simulink model "Basic_DMT"  (R2014b)
settings: Solver=FixedStepDiscrete  SolverMode=SingleTasking  StartTime=0.0  StopTime=25e-6-14e-9*24  RelTol=1e-3
PreLoadFcn:
  | userName = getenv('UserName');
  | 
  | if strcmp(userName,'Tim')
  | cd C:\Users\Tim\Documents\GitHub\MA_1\Basic_DMT
  | else
  | cd C:\Users\Tim-UML\Documents\GitHub\MA_1\Basic_DMT
  | end
InitFcn:
  | userName = getenv('UserName');
  | 
  | if strcmp(userName,'Tim')
  | cd C:\Users\Tim\Documents\GitHub\MA_1\Basic_DMT
  | else
  | cd C:\Users\Tim-UML\Documents\GitHub\MA_1\Basic_DMT
  | end
values from neighbouring files (symbols this model uses):
  a0 = 0.21194908595403703    (= 0.211949085954)    [initScript.m]
  a1 = 0.576101828091926    (= 0.576101828092)    [initScript.m]
  a2 = a0    (= 0.211949085954)    [initScript.m]
  beta = 1    [initScript.m]
  bitPerSymb = 4    [initScript.m]
  chanDownFact = Tchan/SystemPeriod    [initScript.m]
  fftLen = 16    [initScript.m]
  fftLenActive = fftLenDMT    (= 32)    [initScript.m]
  fftLenDMT = 2*fftLen    (= 32)    [initScript.m]
  GI_Active = GI_LenDMT    (= 0)    [initScript.m]
  GI_Len = 0    [initScript.m]
  GI_LenDMT = 0    [initScript.m]
  M = log2(fftLen)    [initScript.m]
  sysgenSystemPeriod = 4e-9    (= 4e-09)    [initScript.m]
  SystemPeriod = 4e-9    (= 4e-09)    [initScript.m]
  upsampleFactor = 1    [initScript.m]
  usedSubCar = 14    [initScript.m]
undefined symbols (not defined in the file or in its folder): bitCount, get, modu_mode, Tb, Ts
libraries: xbsIndex_r4 x822, commdigbbndam3 x59, simulink x42, dspsigops x7, commrandsrc2 x6, dspbuff3 x4, dspxfrm3 x3, dspswit3 x2, commseqgen2 x1, dsparch4 x1, commutil2 x1, dspsnks4 x1
(part 5 of 10)

== system Basic_DMT/Sysgen_AWGN/Yes_AWGN ==
  Re : Inport
  Im : Inport  Port=2
  AddSub : xbsIndex_r4/AddSub  mode=Subtraction  use_carryin=off  use_carryout=off  en=off  latency=1  precision=User Defined  arith_type="Signed  (2's comp)"  n_bits=bitCount+(log2(fftLen)+1)  bin_pt=fracLen  quantization="Round  (unbiased: +/- Inf)"  overflow=Saturate  use_behavioral_HDL=off  hw_selection=Fabric  pipelined=off  dbl_ovrd=off  block_type=addsub
  AddSub1 : xbsIndex_r4/AddSub  mode=Addition  use_carryin=off  use_carryout=off  en=off  latency=0  precision=User Defined  arith_type="Signed  (2's comp)"  n_bits=bitCount+(log2(fftLen)+1)  bin_pt=fracLen  quantization="Round  (unbiased: +/- Inf)"  overflow=Saturate  use_behavioral_HDL=off  hw_selection=Fabric  pipelined=off  dbl_ovrd=off  block_type=addsub
  AddSub2 : xbsIndex_r4/AddSub  mode=Addition  use_carryin=off  use_carryout=off  en=off  latency=0  precision=User Defined  arith_type="Signed  (2's comp)"  n_bits=bitCount+(log2(fftLen)+1)  bin_pt=fracLen  quantization="Round  (unbiased: +/- Inf)"  overflow=Saturate  use_behavioral_HDL=off  hw_selection=Fabric  pipelined=off  dbl_ovrd=off  block_type=addsub
  Assert : xbsIndex_r4/Assert  assert_type=on  type_source=Explicitly  gui_display_data_type=Boolean  arith_type=Boolean  n_bits=16  bin_pt=14  preci_type=Single  exp_width=8  frac_width=24  assert_rate=on  rate_source=Explicitly  period=bitPerSymb*usedSubCar*Ts/(fftLenActive+GI_Active)  output_port=on  block_type=assert
  CMult : xbsIndex_r4/CMult  const=1.58*2  gui_display_data_type=Fixed-point  const_n_bits=bitCount+(log2(fftLen)+1)  const_bin_pt=fracLen  float_type=Single  exp_bits=8  fraction_bits=24  en=off  latency=1  precision=User Defined  arith_type="Signed  (2's comp)"  n_bits=bitCount+(log2(fftLen)+1)  bin_pt=fracLen  quantization="Round  (unbiased: +/- Inf)"  overflow=Saturate  use_behavioral_HDL=off  mem_type=Distributed RAM  pipeline=off  dbl_ovrd=off  block_type=cmult
  Constant1 : xbsIndex_r4/Constant  const=0.5  gui_display_data_type=Fixed-point  arith_type=Signed (2's comp)  n_bits=bitCount+(log2(fftLen)+1)  bin_pt=fracLen  preci_type=Single  exp_width=8  frac_width=24  explicit_period=on  period=bitPerSymb*usedSubCar*Ts/(fftLenActive+GI_Active)  equ=P=C  opselect=C  inp2=PCIN>>17  opr=+  inp1=P  carry=CIN  dbl_ovrd=off  block_type=constant
  Convert : xbsIndex_r4/Convert  gui_display_data_type=Fixed-point  arith_type="Signed  (2's comp)"  n_bits=bitCount+(log2(fftLen)+1)  bin_pt=fracLen  float_type=Single  exp_bits=8  fraction_bits=24  quantization=Truncate  overflow=Wrap  en=off  latency=1  pipeline=off  dbl_ovrd=off  block_type=convert
  Logical : xbsIndex_r4/Logical  logical_function=XOR  inputs=4  en=off  latency=0  precision=Full  arith_type=Unsigned  n_bits=16  bin_pt=0  align_bp=on  dbl_ovrd=off  block_type=logical
  Logical1 : xbsIndex_r4/Logical  logical_function=XOR  inputs=2  en=off  latency=0  precision=Full  arith_type=Unsigned  n_bits=16  bin_pt=0  align_bp=on  dbl_ovrd=off  block_type=logical
  Register{,1..4} (5 alike) : xbsIndex_r4/Register  init=0  rst=off  en=off  dbl_ovrd=off  block_type=register
  Register5 : xbsIndex_r4/Register  init=1  rst=off  en=off  dbl_ovrd=off  block_type=register
  Re_out : Outport
  Im_out : Outport  Port=2
  db_bool : Outport  Port=3
  db_full : Outport  Port=4
  wires:
  Register/1 -> Logical/3, Register2/1
  Register1/1 -> Assert/1
  Register2/1 -> Register3/1
  Register4/1 -> Logical1/2, Register5/1
  Logical/1 -> db_bool/1, Convert/1
  Convert/1 -> AddSub/1
  Constant1/1 -> AddSub/2
  CMult/1 -> db_full/1, AddSub2/2, AddSub1/2
  AddSub/1 -> CMult/1
  Register5/1 -> Logical/1, Logical1/1
  Logical1/1 -> Register1/1
  Register3/1 -> Logical/2, Register4/1
  Assert/1 -> Logical/4, Register/1
  Re/1 -> AddSub1/1
  Im/1 -> AddSub2/1
  AddSub1/1 -> Re_out/1
  AddSub2/1 -> Im_out/1

== system Basic_DMT/Sysgen_Channel/No_channel ==
  Re : Inport
  Im : Inport  Port=2
  Delay : xbsIndex_r4/Delay  rst=off  infoeditControl=Selection of Reset will increase slice count due to use of real FFs and instead of SRLs  en=off  latency=fftLen+GI_Len  reg_retiming=off  dbl_ovrd=off  block_type=delay
  Delay1 : xbsIndex_r4/Delay  rst=off  infoeditControl=Selection of Reset will increase slice count due to use of real FFs and instead of SRLs  en=off  latency=fftLen+GI_Len  reg_retiming=off  dbl_ovrd=off  block_type=delay
  Re_out : Outport
  Im_out : Outport  Port=2
  wires:
  Re/1 -> Delay/1
  Delay/1 -> Re_out/1
  Im/1 -> Delay1/1
  Delay1/1 -> Im_out/1

== system Basic_DMT/Sysgen_Channel/Yes_Channel ==
  Re : Inport
  Im : Inport  Port=2
  AddSub{,1..3} (4 alike) : xbsIndex_r4/AddSub  mode=Addition  use_carryin=off  use_carryout=off  en=off  latency=0  precision=User Defined  arith_type="Signed  (2's comp)"  n_bits=bitCount+(log2(fftLen)+1)  bin_pt=fracLen  quantization="Round  (unbiased: +/- Inf)"  overflow=Saturate  use_behavioral_HDL=off  hw_selection=Fabric  pipelined=off  dbl_ovrd=off  block_type=addsub
  CMult : xbsIndex_r4/CMult  const=a0  gui_display_data_type=Fixed-point  const_n_bits=bitCount+(log2(fftLen)+1)  const_bin_pt=fracLen  float_type=Single  exp_bits=8  fraction_bits=24  en=off  latency=0  precision=User Defined  arith_type="Signed  (2's comp)"  n_bits=bitCount+(log2(fftLen)+1)  bin_pt=fracLen  quantization="Round  (unbiased: +/- Inf)"  overflow=Saturate  use_behavioral_HDL=off  mem_type=Distributed RAM  pipeline=off  dbl_ovrd=off  block_type=cmult
  CMult1 : xbsIndex_r4/CMult  const=a1  gui_display_data_type=Fixed-point  const_n_bits=bitCount+(log2(fftLen)+1)  const_bin_pt=fracLen  float_type=Single  exp_bits=8  fraction_bits=24  en=off  latency=0  precision=User Defined  arith_type="Signed  (2's comp)"  n_bits=bitCount+(log2(fftLen)+1)  bin_pt=fracLen  quantization="Round  (unbiased: +/- Inf)"  overflow=Saturate  use_behavioral_HDL=off  mem_type=Distributed RAM  pipeline=off  dbl_ovrd=off  block_type=cmult
  CMult2 : xbsIndex_r4/CMult  const=a0  gui_display_data_type=Fixed-point  const_n_bits=bitCount+(log2(fftLen)+1)  const_bin_pt=fracLen  float_type=Single  exp_bits=8  fraction_bits=24  en=off  latency=0  precision=User Defined  arith_type="Signed  (2's comp)"  n_bits=bitCount+(log2(fftLen)+1)  bin_pt=fracLen  quantization="Round  (unbiased: +/- Inf)"  overflow=Saturate  use_behavioral_HDL=off  mem_type=Distributed RAM  pipeline=off  dbl_ovrd=off  block_type=cmult
  CMult3 : xbsIndex_r4/CMult  const=a1  gui_display_data_type=Fixed-point  const_n_bits=bitCount+(log2(fftLen)+1)  const_bin_pt=fracLen  float_type=Single  exp_bits=8  fraction_bits=24  en=off  latency=0  precision=User Defined  arith_type="Signed  (2's comp)"  n_bits=bitCount+(log2(fftLen)+1)  bin_pt=fracLen  quantization="Round  (unbiased: +/- Inf)"  overflow=Saturate  use_behavioral_HDL=off  mem_type=Distributed RAM  pipeline=off  dbl_ovrd=off  block_type=cmult
  CMult4 : xbsIndex_r4/CMult  const=a2  gui_display_data_type=Fixed-point  const_n_bits=bitCount+(log2(fftLen)+1)  const_bin_pt=fracLen  float_type=Single  exp_bits=8  fraction_bits=24  en=off  latency=0  precision=User Defined  arith_type="Signed  (2's comp)"  n_bits=bitCount+(log2(fftLen)+1)  bin_pt=fracLen  quantization="Round  (unbiased: +/- Inf)"  overflow=Saturate  use_behavioral_HDL=off  mem_type=Distributed RAM  pipeline=off  dbl_ovrd=off  block_type=cmult
  CMult5 : xbsIndex_r4/CMult  const=a2  gui_display_data_type=Fixed-point  const_n_bits=bitCount+(log2(fftLen)+1)  const_bin_pt=fracLen  float_type=Single  exp_bits=8  fraction_bits=24  en=off  latency=0  precision=User Defined  arith_type="Signed  (2's comp)"  n_bits=bitCount+(log2(fftLen)+1)  bin_pt=fracLen  quantization="Round  (unbiased: +/- Inf)"  overflow=Saturate  use_behavioral_HDL=off  mem_type=Distributed RAM  pipeline=off  dbl_ovrd=off  block_type=cmult
  Delay{,1..3} (4 alike) : xbsIndex_r4/Delay  rst=off  infoeditControl=Selection of Reset will increase slice count due to use of real FFs and instead of SRLs  en=off  latency=1  reg_retiming=off  dbl_ovrd=off  block_type=delay
  Delay4 : xbsIndex_r4/Delay  rst=off  infoeditControl=Selection of Reset will increase slice count due to use of real FFs and instead of SRLs  en=off  latency=fftLen-1+GI_Len  reg_retiming=off  dbl_ovrd=off  block_type=delay
  Delay5 : xbsIndex_r4/Delay  rst=off  infoeditControl=Selection of Reset will increase slice count due to use of real FFs and instead of SRLs  en=off  latency=fftLen-1+GI_Len  reg_retiming=off  dbl_ovrd=off  block_type=delay
  TP_2nd_ord : Subsystem  Commented=on
  Re_out : Outport
  Im_out : Outport  Port=2
  wires:
  CMult1/1 -> AddSub/1
  CMult/1 -> AddSub/2
  Delay/1 -> Delay2/1, CMult1/1
  Re/1 -> CMult/1, Delay/1
  CMult4/1 -> AddSub1/1
  Delay2/1 -> CMult4/1
  AddSub1/1 -> Delay4/1
  Delay4/1 -> Re_out/1
  Delay5/1 -> Im_out/1
  AddSub/1 -> AddSub1/2
  CMult3/1 -> AddSub2/1
  CMult2/1 -> AddSub2/2
  Delay1/1 -> Delay3/1, CMult3/1
  Im/1 -> CMult2/1, Delay1/1
  CMult5/1 -> AddSub3/1
  Delay3/1 -> CMult5/1
  AddSub2/1 -> AddSub3/2
  AddSub3/1 -> Delay5/1

== system Basic_DMT/Sysgen_IFFTaPIS/Guard_Interval ==
  note: 1) Add Subsystem or Model blocks as valid variant choices.
      | 2) You cannot connect blocks at this level. At simulation, connectivity is automatically
      | determined, based on the active variant and port name matching.
  Re_In : Inport
  Im_In : Inport  Port=2
  No_GI : Subsystem  VariantControl=guardInterval==1
  Set_GI_DMT : Subsystem  VariantControl=guardInterval==2&&dmtOfdm==2
  Set_GI_OFDM : Subsystem  VariantControl=guardInterval==2&&dmtOfdm==1
  Re : Outport
  Im : Outport  Port=2

== system Basic_DMT/Sysgen_IFFTaPIS/OFDMorDMT ==
  note: 1) Add Subsystem or Model blocks as valid variant choices.
      | 2) You cannot connect blocks at this level. At simulation, connectivity is automatically
      | determined, based on the active variant and port name matching.
  Re_Sub1 : Inport
  Im_Sub1 : Inport  Port=2
  Re_Sub2 : Inport  Port=3
  Im_Sub2 : Inport  Port=4
  Re_Sub3 : Inport  Port=5
  Im_Sub3 : Inport  Port=6
  Re_Sub4 : Inport  Port=7
  Im_Sub4 : Inport  Port=8
  Re_Sub5 : Inport  Port=9
  Im_Sub5 : Inport  Port=10
  Re_Sub6 : Inport  Port=11
  Im_Sub6 : Inport  Port=12
  Re_Sub7 : Inport  Port=13
  Im_Sub7 : Inport  Port=14
  Re_Sub8 : Inport  Port=15
  Im_Sub8 : Inport  Port=16
  Re_Sub9 : Inport  Port=17
  Im_Sub9 : Inport  Port=18
  Re_Sub10 : Inport  Port=19
  Im_Sub10 : Inport  Port=20
  Re_Sub11 : Inport  Port=21
  Im_Sub11 : Inport  Port=22
  Re_Sub12 : Inport  Port=23
  Im_Sub12 : Inport  Port=24
  Re_Sub13 : Inport  Port=25
  Im_Sub13 : Inport  Port=26
  Re_Sub14 : Inport  Port=27
  Im_Sub14 : Inport  Port=28
  IFFT_DMT : Subsystem  VariantControl=dmtOfdm==2
  IFFT_OFDM : Subsystem  VariantControl=dmtOfdm==1
  Re : Outport
  Im : Outport  Port=2
  Debug_Re : Outport  Port=3
  Debug_Im : Outport  Port=4

== system Basic_DMT/Sysgen_Modulation/16-QAM1 ==
  In1 : Inport
  BitBasher : xbsIndex_r4/BitBasher  bitexpr=|  display_expr=on  sr_1=b  arith_type1=Unsigned  bin_pt1=0  sr_2=c  arith_type2=Unsigned  bin_pt2=0  sr_3=3  arith_type3=Unsigned  bin_pt3=0  sr_4=4  arith_type4=Unsigned  bin_pt4=0  dbl_ovrd=off  block_type=bitbasher
      | b={a[3:2]}
      | c={a[1:0]}
  Constant1 : xbsIndex_r4/Constant  const=-3  gui_display_data_type=Fixed-point  arith_type=Signed (2's comp)  n_bits=bitCount  bin_pt=fracLen  preci_type=Single  exp_width=8  frac_width=24  explicit_period=on  period=Ts*usedSubCar* bitPerSymb  equ=P=C  opselect=C  inp2=PCIN>>17  opr=+  inp1=P  carry=CIN  dbl_ovrd=off  block_type=constant
  Constant2 : xbsIndex_r4/Constant  const=-1  gui_display_data_type=Fixed-point  arith_type=Signed (2's comp)  n_bits=bitCount  bin_pt=fracLen  preci_type=Single  exp_width=8  frac_width=24  explicit_period=on  period=Ts*usedSubCar* bitPerSymb  equ=P=C  opselect=C  inp2=PCIN>>17  opr=+  inp1=P  carry=CIN  dbl_ovrd=off  block_type=constant
  Constant3 : xbsIndex_r4/Constant  const=3  gui_display_data_type=Fixed-point  arith_type=Signed (2's comp)  n_bits=bitCount  bin_pt=fracLen  preci_type=Single  exp_width=8  frac_width=24  explicit_period=on  period=Ts*usedSubCar* bitPerSymb  equ=P=C  opselect=C  inp2=PCIN>>17  opr=+  inp1=P  carry=CIN  dbl_ovrd=off  block_type=constant
  Constant4 : xbsIndex_r4/Constant  const=1  gui_display_data_type=Fixed-point  arith_type=Signed (2's comp)  n_bits=bitCount  bin_pt=fracLen  preci_type=Single  exp_width=8  frac_width=24  explicit_period=on  period=Ts*usedSubCar* bitPerSymb  equ=P=C  opselect=C  inp2=PCIN>>17  opr=+  inp1=P  carry=CIN  dbl_ovrd=off  block_type=constant
  Constant5 : xbsIndex_r4/Constant  const=1  gui_display_data_type=Fixed-point  arith_type=Signed (2's comp)  n_bits=bitCount  bin_pt=fracLen  preci_type=Single  exp_width=8  frac_width=24  explicit_period=on  period=Ts*usedSubCar* bitPerSymb  equ=P=C  opselect=C  inp2=PCIN>>17  opr=+  inp1=P  carry=CIN  dbl_ovrd=off  block_type=constant
  Constant6 : xbsIndex_r4/Constant  const=-3  gui_display_data_type=Fixed-point  arith_type=Signed (2's comp)  n_bits=bitCount  bin_pt=fracLen  preci_type=Single  exp_width=8  frac_width=24  explicit_period=on  period=Ts*usedSubCar* bitPerSymb  equ=P=C  opselect=C  inp2=PCIN>>17  opr=+  inp1=P  carry=CIN  dbl_ovrd=off  block_type=constant
  Constant7 : xbsIndex_r4/Constant  const=-1  gui_display_data_type=Fixed-point  arith_type=Signed (2's comp)  n_bits=bitCount  bin_pt=fracLen  preci_type=Single  exp_width=8  frac_width=24  explicit_period=on  period=Ts*usedSubCar* bitPerSymb  equ=P=C  opselect=C  inp2=PCIN>>17  opr=+  inp1=P  carry=CIN  dbl_ovrd=off  block_type=constant
  Constant9 : xbsIndex_r4/Constant  const=3  gui_display_data_type=Fixed-point  arith_type=Signed (2's comp)  n_bits=bitCount  bin_pt=fracLen  preci_type=Single  exp_width=8  frac_width=24  explicit_period=on  period=Ts*usedSubCar* bitPerSymb  equ=P=C  opselect=C  inp2=PCIN>>17  opr=+  inp1=P  carry=CIN  dbl_ovrd=off  block_type=constant
  Mux : xbsIndex_r4/Mux  inputs=4  en=off  latency=1  precision=Full  arith_type=Unsigned  n_bits=16  bin_pt=14  quantization=Truncate  overflow=Wrap  dbl_ovrd=off  block_type=mux
  Mux1 : xbsIndex_r4/Mux  inputs=4  en=off  latency=1  precision=Full  arith_type=Unsigned  n_bits=16  bin_pt=14  quantization=Truncate  overflow=Wrap  dbl_ovrd=off  block_type=mux
  Out2 : Outport
  Out3 : Outport  Port=2
  wires:
  Mux1/1 -> Out3/1
  In1/1 -> BitBasher/1
  Constant1/1 -> Mux/2
  Constant2/1 -> Mux/3
  BitBasher/1 -> Mux/1
  Constant9/1 -> Mux1/2
  Constant5/1 -> Mux1/3
  Constant7/1 -> Mux1/5
  Constant6/1 -> Mux1/4
  BitBasher/2 -> Mux1/1
  Constant4/1 -> Mux/5
  Mux/1 -> Out2/1
  Constant3/1 -> Mux/4

== system Basic_DMT/Sysgen_Modulation/16-QAM10 ==
  In1 : Inport
  BitBasher : xbsIndex_r4/BitBasher  bitexpr=|  display_expr=on  sr_1=b  arith_type1=Unsigned  bin_pt1=0  sr_2=c  arith_type2=Unsigned  bin_pt2=0  sr_3=3  arith_type3=Unsigned  bin_pt3=0  sr_4=4  arith_type4=Unsigned  bin_pt4=0  dbl_ovrd=off  block_type=bitbasher
      | b={a[3:2]}
      | c={a[1:0]}
  Constant1 : xbsIndex_r4/Constant  const=-3  gui_display_data_type=Fixed-point  arith_type=Signed (2's comp)  n_bits=bitCount  bin_pt=fracLen  preci_type=Single  exp_width=8  frac_width=24  explicit_period=on  period=Ts*usedSubCar* bitPerSymb  equ=P=C  opselect=C  inp2=PCIN>>17  opr=+  inp1=P  carry=CIN  dbl_ovrd=off  block_type=constant
  Constant2 : xbsIndex_r4/Constant  const=-1  gui_display_data_type=Fixed-point  arith_type=Signed (2's comp)  n_bits=bitCount  bin_pt=fracLen  preci_type=Single  exp_width=8  frac_width=24  explicit_period=on  period=Ts*usedSubCar* bitPerSymb  equ=P=C  opselect=C  inp2=PCIN>>17  opr=+  inp1=P  carry=CIN  dbl_ovrd=off  block_type=constant
  Constant3 : xbsIndex_r4/Constant  const=3  gui_display_data_type=Fixed-point  arith_type=Signed (2's comp)  n_bits=bitCount  bin_pt=fracLen  preci_type=Single  exp_width=8  frac_width=24  explicit_period=on  period=Ts*usedSubCar* bitPerSymb  equ=P=C  opselect=C  inp2=PCIN>>17  opr=+  inp1=P  carry=CIN  dbl_ovrd=off  block_type=constant
  Constant4 : xbsIndex_r4/Constant  const=1  gui_display_data_type=Fixed-point  arith_type=Signed (2's comp)  n_bits=bitCount  bin_pt=fracLen  preci_type=Single  exp_width=8  frac_width=24  explicit_period=on  period=Ts*usedSubCar* bitPerSymb  equ=P=C  opselect=C  inp2=PCIN>>17  opr=+  inp1=P  carry=CIN  dbl_ovrd=off  block_type=constant
  Constant5 : xbsIndex_r4/Constant  const=1  gui_display_data_type=Fixed-point  arith_type=Signed (2's comp)  n_bits=bitCount  bin_pt=fracLen  preci_type=Single  exp_width=8  frac_width=24  explicit_period=on  period=Ts*usedSubCar* bitPerSymb  equ=P=C  opselect=C  inp2=PCIN>>17  opr=+  inp1=P  carry=CIN  dbl_ovrd=off  block_type=constant
  Constant6 : xbsIndex_r4/Constant  const=-3  gui_display_data_type=Fixed-point  arith_type=Signed (2's comp)  n_bits=bitCount  bin_pt=fracLen  preci_type=Single  exp_width=8  frac_width=24  explicit_period=on  period=Ts*usedSubCar* bitPerSymb  equ=P=C  opselect=C  inp2=PCIN>>17  opr=+  inp1=P  carry=CIN  dbl_ovrd=off  block_type=constant
  Constant7 : xbsIndex_r4/Constant  const=-1  gui_display_data_type=Fixed-point  arith_type=Signed (2's comp)  n_bits=bitCount  bin_pt=fracLen  preci_type=Single  exp_width=8  frac_width=24  explicit_period=on  period=Ts*usedSubCar* bitPerSymb  equ=P=C  opselect=C  inp2=PCIN>>17  opr=+  inp1=P  carry=CIN  dbl_ovrd=off  block_type=constant
  Constant9 : xbsIndex_r4/Constant  const=3  gui_display_data_type=Fixed-point  arith_type=Signed (2's comp)  n_bits=bitCount  bin_pt=fracLen  preci_type=Single  exp_width=8  frac_width=24  explicit_period=on  period=Ts*usedSubCar* bitPerSymb  equ=P=C  opselect=C  inp2=PCIN>>17  opr=+  inp1=P  carry=CIN  dbl_ovrd=off  block_type=constant
  Mux : xbsIndex_r4/Mux  inputs=4  en=off  latency=1  precision=Full  arith_type=Unsigned  n_bits=16  bin_pt=14  quantization=Truncate  overflow=Wrap  dbl_ovrd=off  block_type=mux
  Mux1 : xbsIndex_r4/Mux  inputs=4  en=off  latency=1  precision=Full  arith_type=Unsigned  n_bits=16  bin_pt=14  quantization=Truncate  overflow=Wrap  dbl_ovrd=off  block_type=mux
  Out2 : Outport
  Out3 : Outport  Port=2
  wires:
  Mux1/1 -> Out3/1
  In1/1 -> BitBasher/1
  Constant1/1 -> Mux/2
  Constant2/1 -> Mux/3
  BitBasher/1 -> Mux/1
  Constant9/1 -> Mux1/2
  Constant5/1 -> Mux1/3
  Constant7/1 -> Mux1/5
  Constant6/1 -> Mux1/4
  BitBasher/2 -> Mux1/1
  Constant4/1 -> Mux/5
  Mux/1 -> Out2/1
  Constant3/1 -> Mux/4

== system Basic_DMT/Sysgen_Modulation/16-QAM11 ==
  In1 : Inport
  BitBasher : xbsIndex_r4/BitBasher  bitexpr=|  display_expr=on  sr_1=b  arith_type1=Unsigned  bin_pt1=0  sr_2=c  arith_type2=Unsigned  bin_pt2=0  sr_3=3  arith_type3=Unsigned  bin_pt3=0  sr_4=4  arith_type4=Unsigned  bin_pt4=0  dbl_ovrd=off  block_type=bitbasher
      | b={a[3:2]}
      | c={a[1:0]}
  Constant1 : xbsIndex_r4/Constant  const=-3  gui_display_data_type=Fixed-point  arith_type=Signed (2's comp)  n_bits=bitCount  bin_pt=fracLen  preci_type=Single  exp_width=8  frac_width=24  explicit_period=on  period=Ts*usedSubCar* bitPerSymb  equ=P=C  opselect=C  inp2=PCIN>>17  opr=+  inp1=P  carry=CIN  dbl_ovrd=off  block_type=constant
  Constant2 : xbsIndex_r4/Constant  const=-1  gui_display_data_type=Fixed-point  arith_type=Signed (2's comp)  n_bits=bitCount  bin_pt=fracLen  preci_type=Single  exp_width=8  frac_width=24  explicit_period=on  period=Ts*usedSubCar* bitPerSymb  equ=P=C  opselect=C  inp2=PCIN>>17  opr=+  inp1=P  carry=CIN  dbl_ovrd=off  block_type=constant
  Constant3 : xbsIndex_r4/Constant  const=3  gui_display_data_type=Fixed-point  arith_type=Signed (2's comp)  n_bits=bitCount  bin_pt=fracLen  preci_type=Single  exp_width=8  frac_width=24  explicit_period=on  period=Ts*usedSubCar* bitPerSymb  equ=P=C  opselect=C  inp2=PCIN>>17  opr=+  inp1=P  carry=CIN  dbl_ovrd=off  block_type=constant
  Constant4 : xbsIndex_r4/Constant  const=1  gui_display_data_type=Fixed-point  arith_type=Signed (2's comp)  n_bits=bitCount  bin_pt=fracLen  preci_type=Single  exp_width=8  frac_width=24  explicit_period=on  period=Ts*usedSubCar* bitPerSymb  equ=P=C  opselect=C  inp2=PCIN>>17  opr=+  inp1=P  carry=CIN  dbl_ovrd=off  block_type=constant
  Constant5 : xbsIndex_r4/Constant  const=1  gui_display_data_type=Fixed-point  arith_type=Signed (2's comp)  n_bits=bitCount  bin_pt=fracLen  preci_type=Single  exp_width=8  frac_width=24  explicit_period=on  period=Ts*usedSubCar* bitPerSymb  equ=P=C  opselect=C  inp2=PCIN>>17  opr=+  inp1=P  carry=CIN  dbl_ovrd=off  block_type=constant
  Constant6 : xbsIndex_r4/Constant  const=-3  gui_display_data_type=Fixed-point  arith_type=Signed (2's comp)  n_bits=bitCount  bin_pt=fracLen  preci_type=Single  exp_width=8  frac_width=24  explicit_period=on  period=Ts*usedSubCar* bitPerSymb  equ=P=C  opselect=C  inp2=PCIN>>17  opr=+  inp1=P  carry=CIN  dbl_ovrd=off  block_type=constant
  Constant7 : xbsIndex_r4/Constant  const=-1  gui_display_data_type=Fixed-point  arith_type=Signed (2's comp)  n_bits=bitCount  bin_pt=fracLen  preci_type=Single  exp_width=8  frac_width=24  explicit_period=on  period=Ts*usedSubCar* bitPerSymb  equ=P=C  opselect=C  inp2=PCIN>>17  opr=+  inp1=P  carry=CIN  dbl_ovrd=off  block_type=constant
  Constant9 : xbsIndex_r4/Constant  const=3  gui_display_data_type=Fixed-point  arith_type=Signed (2's comp)  n_bits=bitCount  bin_pt=fracLen  preci_type=Single  exp_width=8  frac_width=24  explicit_period=on  period=Ts*usedSubCar* bitPerSymb  equ=P=C  opselect=C  inp2=PCIN>>17  opr=+  inp1=P  carry=CIN  dbl_ovrd=off  block_type=constant
  Mux : xbsIndex_r4/Mux  inputs=4  en=off  latency=1  precision=Full  arith_type=Unsigned  n_bits=16  bin_pt=14  quantization=Truncate  overflow=Wrap  dbl_ovrd=off  block_type=mux
  Mux1 : xbsIndex_r4/Mux  inputs=4  en=off  latency=1  precision=Full  arith_type=Unsigned  n_bits=16  bin_pt=14  quantization=Truncate  overflow=Wrap  dbl_ovrd=off  block_type=mux
  Out2 : Outport
  Out3 : Outport  Port=2
  wires:
  Mux1/1 -> Out3/1
  In1/1 -> BitBasher/1
  Constant1/1 -> Mux/2
  Constant2/1 -> Mux/3
  BitBasher/1 -> Mux/1
  Constant9/1 -> Mux1/2
  Constant5/1 -> Mux1/3
  Constant7/1 -> Mux1/5
  Constant6/1 -> Mux1/4
  BitBasher/2 -> Mux1/1
  Constant4/1 -> Mux/5
  Mux/1 -> Out2/1
  Constant3/1 -> Mux/4

== system Basic_DMT/Sysgen_Modulation/16-QAM1111 ==
  Inp : Inport
  BitBasher : xbsIndex_r4/BitBasher  bitexpr=|  display_expr=on  sr_1=b  arith_type1=Unsigned  bin_pt1=0  sr_2=c  arith_type2=Unsigned  bin_pt2=0  sr_3=3  arith_type3=Unsigned  bin_pt3=0  sr_4=4  arith_type4=Unsigned  bin_pt4=0  dbl_ovrd=off  block_type=bitbasher
      | b={a[3:2]}
      | c={a[1:0]}
  Constant1 : xbsIndex_r4/Constant  const=-3  gui_display_data_type=Floating-point  arith_type=Signed (2's comp)  n_bits=16  bin_pt=12  preci_type=Single  exp_width=8  frac_width=24  explicit_period=off  period=Ts  equ=P=C  opselect=C  inp2=PCIN>>17  opr=+  inp1=P  carry=CIN  dbl_ovrd=off  block_type=constant
  Constant2 : xbsIndex_r4/Constant  const=-1  gui_display_data_type=Floating-point  arith_type=Signed (2's comp)  n_bits=16  bin_pt=12  preci_type=Single  exp_width=8  frac_width=24  explicit_period=off  period=Ts  equ=P=C  opselect=C  inp2=PCIN>>17  opr=+  inp1=P  carry=CIN  dbl_ovrd=off  block_type=constant
  Constant3 : xbsIndex_r4/Constant  const=3  gui_display_data_type=Floating-point  arith_type=Signed (2's comp)  n_bits=16  bin_pt=12  preci_type=Single  exp_width=8  frac_width=24  explicit_period=off  period=Ts  equ=P=C  opselect=C  inp2=PCIN>>17  opr=+  inp1=P  carry=CIN  dbl_ovrd=off  block_type=constant
  Constant4 : xbsIndex_r4/Constant  const=1  gui_display_data_type=Floating-point  arith_type=Signed (2's comp)  n_bits=16  bin_pt=12  preci_type=Single  exp_width=8  frac_width=24  explicit_period=off  period=Ts  equ=P=C  opselect=C  inp2=PCIN>>17  opr=+  inp1=P  carry=CIN  dbl_ovrd=off  block_type=constant
  Constant5 : xbsIndex_r4/Constant  const=3  gui_display_data_type=Floating-point  arith_type=Signed (2's comp)  n_bits=16  bin_pt=12  preci_type=Single  exp_width=8  frac_width=24  explicit_period=off  period=Ts  equ=P=C  opselect=C  inp2=PCIN>>17  opr=+  inp1=P  carry=CIN  dbl_ovrd=off  block_type=constant
  Constant6 : xbsIndex_r4/Constant  const=1  gui_display_data_type=Floating-point  arith_type=Signed (2's comp)  n_bits=16  bin_pt=12  preci_type=Single  exp_width=8  frac_width=24  explicit_period=off  period=Ts  equ=P=C  opselect=C  inp2=PCIN>>17  opr=+  inp1=P  carry=CIN  dbl_ovrd=off  block_type=constant
  Constant7 : xbsIndex_r4/Constant  const=-3  gui_display_data_type=Floating-point  arith_type=Signed (2's comp)  n_bits=16  bin_pt=12  preci_type=Single  exp_width=8  frac_width=24  explicit_period=off  period=Ts  equ=P=C  opselect=C  inp2=PCIN>>17  opr=+  inp1=P  carry=CIN  dbl_ovrd=off  block_type=constant
  Constant8 : xbsIndex_r4/Constant  const=-1  gui_display_data_type=Floating-point  arith_type=Signed (2's comp)  n_bits=16  bin_pt=12  preci_type=Single  exp_width=8  frac_width=24  explicit_period=off  period=Ts  equ=P=C  opselect=C  inp2=PCIN>>17  opr=+  inp1=P  carry=CIN  dbl_ovrd=off  block_type=constant
  Mux : xbsIndex_r4/Mux  inputs=4  en=off  latency=1  precision=Full  arith_type=Unsigned  n_bits=16  bin_pt=14  quantization=Truncate  overflow=Wrap  dbl_ovrd=off  block_type=mux
  Mux1 : xbsIndex_r4/Mux  inputs=4  en=off  latency=1  precision=Full  arith_type=Unsigned  n_bits=16  bin_pt=14  quantization=Truncate  overflow=Wrap  dbl_ovrd=off  block_type=mux
  Re : Outport
  Im : Outport  Port=2
  wires:
  Mux1/1 -> Im/1
  Inp/1 -> BitBasher/1
  Constant1/1 -> Mux/2
  Constant2/1 -> Mux/3
  BitBasher/1 -> Mux/1
  Constant5/1 -> Mux1/2
  Constant6/1 -> Mux1/3
  Constant8/1 -> Mux1/5
  Constant7/1 -> Mux1/4
  BitBasher/2 -> Mux1/1
  Constant4/1 -> Mux/5
  Mux/1 -> Re/1
  Constant3/1 -> Mux/4

== system Basic_DMT/Sysgen_Modulation/16-QAM12 ==
  In1 : Inport
  BitBasher : xbsIndex_r4/BitBasher  bitexpr=|  display_expr=on  sr_1=b  arith_type1=Unsigned  bin_pt1=0  sr_2=c  arith_type2=Unsigned  bin_pt2=0  sr_3=3  arith_type3=Unsigned  bin_pt3=0  sr_4=4  arith_type4=Unsigned  bin_pt4=0  dbl_ovrd=off  block_type=bitbasher
      | b={a[3:2]}
      | c={a[1:0]}
  Constant1 : xbsIndex_r4/Constant  const=-3  gui_display_data_type=Fixed-point  arith_type=Signed (2's comp)  n_bits=bitCount  bin_pt=fracLen  preci_type=Single  exp_width=8  frac_width=24  explicit_period=on  period=Ts*usedSubCar* bitPerSymb  equ=P=C  opselect=C  inp2=PCIN>>17  opr=+  inp1=P  carry=CIN  dbl_ovrd=off  block_type=constant
  Constant2 : xbsIndex_r4/Constant  const=-1  gui_display_data_type=Fixed-point  arith_type=Signed (2's comp)  n_bits=bitCount  bin_pt=fracLen  preci_type=Single  exp_width=8  frac_width=24  explicit_period=on  period=Ts*usedSubCar* bitPerSymb  equ=P=C  opselect=C  inp2=PCIN>>17  opr=+  inp1=P  carry=CIN  dbl_ovrd=off  block_type=constant
  Constant3 : xbsIndex_r4/Constant  const=3  gui_display_data_type=Fixed-point  arith_type=Signed (2's comp)  n_bits=bitCount  bin_pt=fracLen  preci_type=Single  exp_width=8  frac_width=24  explicit_period=on  period=Ts*usedSubCar* bitPerSymb  equ=P=C  opselect=C  inp2=PCIN>>17  opr=+  inp1=P  carry=CIN  dbl_ovrd=off  block_type=constant
  Constant4 : xbsIndex_r4/Constant  const=1  gui_display_data_type=Fixed-point  arith_type=Signed (2's comp)  n_bits=bitCount  bin_pt=fracLen  preci_type=Single  exp_width=8  frac_width=24  explicit_period=on  period=Ts*usedSubCar* bitPerSymb  equ=P=C  opselect=C  inp2=PCIN>>17  opr=+  inp1=P  carry=CIN  dbl_ovrd=off  block_type=constant
  Constant5 : xbsIndex_r4/Constant  const=1  gui_display_data_type=Fixed-point  arith_type=Signed (2's comp)  n_bits=bitCount  bin_pt=fracLen  preci_type=Single  exp_width=8  frac_width=24  explicit_period=on  period=Ts*usedSubCar* bitPerSymb  equ=P=C  opselect=C  inp2=PCIN>>17  opr=+  inp1=P  carry=CIN  dbl_ovrd=off  block_type=constant
  Constant6 : xbsIndex_r4/Constant  const=-3  gui_display_data_type=Fixed-point  arith_type=Signed (2's comp)  n_bits=bitCount  bin_pt=fracLen  preci_type=Single  exp_width=8  frac_width=24  explicit_period=on  period=Ts*usedSubCar* bitPerSymb  equ=P=C  opselect=C  inp2=PCIN>>17  opr=+  inp1=P  carry=CIN  dbl_ovrd=off  block_type=constant
  Constant7 : xbsIndex_r4/Constant  const=-1  gui_display_data_type=Fixed-point  arith_type=Signed (2's comp)  n_bits=bitCount  bin_pt=fracLen  preci_type=Single  exp_width=8  frac_width=24  explicit_period=on  period=Ts*usedSubCar* bitPerSymb  equ=P=C  opselect=C  inp2=PCIN>>17  opr=+  inp1=P  carry=CIN  dbl_ovrd=off  block_type=constant
  Constant9 : xbsIndex_r4/Constant  const=3  gui_display_data_type=Fixed-point  arith_type=Signed (2's comp)  n_bits=bitCount  bin_pt=fracLen  preci_type=Single  exp_width=8  frac_width=24  explicit_period=on  period=Ts*usedSubCar* bitPerSymb  equ=P=C  opselect=C  inp2=PCIN>>17  opr=+  inp1=P  carry=CIN  dbl_ovrd=off  block_type=constant
  Mux : xbsIndex_r4/Mux  inputs=4  en=off  latency=1  precision=Full  arith_type=Unsigned  n_bits=16  bin_pt=14  quantization=Truncate  overflow=Wrap  dbl_ovrd=off  block_type=mux
  Mux1 : xbsIndex_r4/Mux  inputs=4  en=off  latency=1  precision=Full  arith_type=Unsigned  n_bits=16  bin_pt=14  quantization=Truncate  overflow=Wrap  dbl_ovrd=off  block_type=mux
  Out2 : Outport
  Out3 : Outport  Port=2
  wires:
  Mux1/1 -> Out3/1
  In1/1 -> BitBasher/1
  Constant1/1 -> Mux/2
  Constant2/1 -> Mux/3
  BitBasher/1 -> Mux/1
  Constant9/1 -> Mux1/2
  Constant5/1 -> Mux1/3
  Constant7/1 -> Mux1/5
  Constant6/1 -> Mux1/4
  BitBasher/2 -> Mux1/1
  Constant4/1 -> Mux/5
  Mux/1 -> Out2/1
  Constant3/1 -> Mux/4

== system Basic_DMT/Sysgen_Modulation/16-QAM13 ==
  In1 : Inport
  BitBasher : xbsIndex_r4/BitBasher  bitexpr=|  display_expr=on  sr_1=b  arith_type1=Unsigned  bin_pt1=0  sr_2=c  arith_type2=Unsigned  bin_pt2=0  sr_3=3  arith_type3=Unsigned  bin_pt3=0  sr_4=4  arith_type4=Unsigned  bin_pt4=0  dbl_ovrd=off  block_type=bitbasher
      | b={a[3:2]}
      | c={a[1:0]}
  Constant1 : xbsIndex_r4/Constant  const=-3  gui_display_data_type=Fixed-point  arith_type=Signed (2's comp)  n_bits=bitCount  bin_pt=fracLen  preci_type=Single  exp_width=8  frac_width=24  explicit_period=on  period=Ts*usedSubCar* bitPerSymb  equ=P=C  opselect=C  inp2=PCIN>>17  opr=+  inp1=P  carry=CIN  dbl_ovrd=off  block_type=constant
  Constant2 : xbsIndex_r4/Constant  const=-1  gui_display_data_type=Fixed-point  arith_type=Signed (2's comp)  n_bits=bitCount  bin_pt=fracLen  preci_type=Single  exp_width=8  frac_width=24  explicit_period=on  period=Ts*usedSubCar* bitPerSymb  equ=P=C  opselect=C  inp2=PCIN>>17  opr=+  inp1=P  carry=CIN  dbl_ovrd=off  block_type=constant
  Constant3 : xbsIndex_r4/Constant  const=3  gui_display_data_type=Fixed-point  arith_type=Signed (2's comp)  n_bits=bitCount  bin_pt=fracLen  preci_type=Single  exp_width=8  frac_width=24  explicit_period=on  period=Ts*usedSubCar* bitPerSymb  equ=P=C  opselect=C  inp2=PCIN>>17  opr=+  inp1=P  carry=CIN  dbl_ovrd=off  block_type=constant
  Constant4 : xbsIndex_r4/Constant  const=1  gui_display_data_type=Fixed-point  arith_type=Signed (2's comp)  n_bits=bitCount  bin_pt=fracLen  preci_type=Single  exp_width=8  frac_width=24  explicit_period=on  period=Ts*usedSubCar* bitPerSymb  equ=P=C  opselect=C  inp2=PCIN>>17  opr=+  inp1=P  carry=CIN  dbl_ovrd=off  block_type=constant
  Constant5 : xbsIndex_r4/Constant  const=1  gui_display_data_type=Fixed-point  arith_type=Signed (2's comp)  n_bits=bitCount  bin_pt=fracLen  preci_type=Single  exp_width=8  frac_width=24  explicit_period=on  period=Ts*usedSubCar* bitPerSymb  equ=P=C  opselect=C  inp2=PCIN>>17  opr=+  inp1=P  carry=CIN  dbl_ovrd=off  block_type=constant
  Constant6 : xbsIndex_r4/Constant  const=-3  gui_display_data_type=Fixed-point  arith_type=Signed (2's comp)  n_bits=bitCount  bin_pt=fracLen  preci_type=Single  exp_width=8  frac_width=24  explicit_period=on  period=Ts*usedSubCar* bitPerSymb  equ=P=C  opselect=C  inp2=PCIN>>17  opr=+  inp1=P  carry=CIN  dbl_ovrd=off  block_type=constant
  Constant7 : xbsIndex_r4/Constant  const=-1  gui_display_data_type=Fixed-point  arith_type=Signed (2's comp)  n_bits=bitCount  bin_pt=fracLen  preci_type=Single  exp_width=8  frac_width=24  explicit_period=on  period=Ts*usedSubCar* bitPerSymb  equ=P=C  opselect=C  inp2=PCIN>>17  opr=+  inp1=P  carry=CIN  dbl_ovrd=off  block_type=constant
  Constant9 : xbsIndex_r4/Constant  const=3  gui_display_data_type=Fixed-point  arith_type=Signed (2's comp)  n_bits=bitCount  bin_pt=fracLen  preci_type=Single  exp_width=8  frac_width=24  explicit_period=on  period=Ts*usedSubCar* bitPerSymb  equ=P=C  opselect=C  inp2=PCIN>>17  opr=+  inp1=P  carry=CIN  dbl_ovrd=off  block_type=constant
  Mux : xbsIndex_r4/Mux  inputs=4  en=off  latency=1  precision=Full  arith_type=Unsigned  n_bits=16  bin_pt=14  quantization=Truncate  overflow=Wrap  dbl_ovrd=off  block_type=mux
  Mux1 : xbsIndex_r4/Mux  inputs=4  en=off  latency=1  precision=Full  arith_type=Unsigned  n_bits=16  bin_pt=14  quantization=Truncate  overflow=Wrap  dbl_ovrd=off  block_type=mux
  Out2 : Outport
  Out3 : Outport  Port=2
  wires:
  Mux1/1 -> Out3/1
  In1/1 -> BitBasher/1
  Constant1/1 -> Mux/2
  Constant2/1 -> Mux/3
  BitBasher/1 -> Mux/1
  Constant9/1 -> Mux1/2
  Constant5/1 -> Mux1/3
  Constant7/1 -> Mux1/5
  Constant6/1 -> Mux1/4
  BitBasher/2 -> Mux1/1
  Constant4/1 -> Mux/5
  Mux/1 -> Out2/1
  Constant3/1 -> Mux/4

== system Basic_DMT/Sysgen_Modulation/16-QAM14 ==
  In1 : Inport
  BitBasher : xbsIndex_r4/BitBasher  bitexpr=|  display_expr=on  sr_1=b  arith_type1=Unsigned  bin_pt1=0  sr_2=c  arith_type2=Unsigned  bin_pt2=0  sr_3=3  arith_type3=Unsigned  bin_pt3=0  sr_4=4  arith_type4=Unsigned  bin_pt4=0  dbl_ovrd=off  block_type=bitbasher
      | b={a[3:2]}
      | c={a[1:0]}
  Constant1 : xbsIndex_r4/Constant  const=-3  gui_display_data_type=Fixed-point  arith_type=Signed (2's comp)  n_bits=bitCount  bin_pt=fracLen  preci_type=Single  exp_width=8  frac_width=24  explicit_period=on  period=Ts*usedSubCar* bitPerSymb  equ=P=C  opselect=C  inp2=PCIN>>17  opr=+  inp1=P  carry=CIN  dbl_ovrd=off  block_type=constant
  Constant2 : xbsIndex_r4/Constant  const=-1  gui_display_data_type=Fixed-point  arith_type=Signed (2's comp)  n_bits=bitCount  bin_pt=fracLen  preci_type=Single  exp_width=8  frac_width=24  explicit_period=on  period=Ts*usedSubCar* bitPerSymb  equ=P=C  opselect=C  inp2=PCIN>>17  opr=+  inp1=P  carry=CIN  dbl_ovrd=off  block_type=constant
  Constant3 : xbsIndex_r4/Constant  const=3  gui_display_data_type=Fixed-point  arith_type=Signed (2's comp)  n_bits=bitCount  bin_pt=fracLen  preci_type=Single  exp_width=8  frac_width=24  explicit_period=on  period=Ts*usedSubCar* bitPerSymb  equ=P=C  opselect=C  inp2=PCIN>>17  opr=+  inp1=P  carry=CIN  dbl_ovrd=off  block_type=constant
  Constant4 : xbsIndex_r4/Constant  const=1  gui_display_data_type=Fixed-point  arith_type=Signed (2's comp)  n_bits=bitCount  bin_pt=fracLen  preci_type=Single  exp_width=8  frac_width=24  explicit_period=on  period=Ts*usedSubCar* bitPerSymb  equ=P=C  opselect=C  inp2=PCIN>>17  opr=+  inp1=P  carry=CIN  dbl_ovrd=off  block_type=constant
  Constant5 : xbsIndex_r4/Constant  const=1  gui_display_data_type=Fixed-point  arith_type=Signed (2's comp)  n_bits=bitCount  bin_pt=fracLen  preci_type=Single  exp_width=8  frac_width=24  explicit_period=on  period=Ts*usedSubCar* bitPerSymb  equ=P=C  opselect=C  inp2=PCIN>>17  opr=+  inp1=P  carry=CIN  dbl_ovrd=off  block_type=constant
  Constant6 : xbsIndex_r4/Constant  const=-3  gui_display_data_type=Fixed-point  arith_type=Signed (2's comp)  n_bits=bitCount  bin_pt=fracLen  preci_type=Single  exp_width=8  frac_width=24  explicit_period=on  period=Ts*usedSubCar* bitPerSymb  equ=P=C  opselect=C  inp2=PCIN>>17  opr=+  inp1=P  carry=CIN  dbl_ovrd=off  block_type=constant
  Constant7 : xbsIndex_r4/Constant  const=-1  gui_display_data_type=Fixed-point  arith_type=Signed (2's comp)  n_bits=bitCount  bin_pt=fracLen  preci_type=Single  exp_width=8  frac_width=24  explicit_period=on  period=Ts*usedSubCar* bitPerSymb  equ=P=C  opselect=C  inp2=PCIN>>17  opr=+  inp1=P  carry=CIN  dbl_ovrd=off  block_type=constant
  Constant9 : xbsIndex_r4/Constant  const=3  gui_display_data_type=Fixed-point  arith_type=Signed (2's comp)  n_bits=bitCount  bin_pt=fracLen  preci_type=Single  exp_width=8  frac_width=24  explicit_period=on  period=Ts*usedSubCar* bitPerSymb  equ=P=C  opselect=C  inp2=PCIN>>17  opr=+  inp1=P  carry=CIN  dbl_ovrd=off  block_type=constant
  Mux : xbsIndex_r4/Mux  inputs=4  en=off  latency=1  precision=Full  arith_type=Unsigned  n_bits=16  bin_pt=14  quantization=Truncate  overflow=Wrap  dbl_ovrd=off  block_type=mux
  Mux1 : xbsIndex_r4/Mux  inputs=4  en=off  latency=1  precision=Full  arith_type=Unsigned  n_bits=16  bin_pt=14  quantization=Truncate  overflow=Wrap  dbl_ovrd=off  block_type=mux
  Out2 : Outport
  Out3 : Outport  Port=2
  wires:
  Mux1/1 -> Out3/1
  In1/1 -> BitBasher/1
  Constant1/1 -> Mux/2
  Constant2/1 -> Mux/3
  BitBasher/1 -> Mux/1
  Constant9/1 -> Mux1/2
  Constant5/1 -> Mux1/3
  Constant7/1 -> Mux1/5
  Constant6/1 -> Mux1/4
  BitBasher/2 -> Mux1/1
  Constant4/1 -> Mux/5
  Mux/1 -> Out2/1
  Constant3/1 -> Mux/4

== system Basic_DMT/Sysgen_Modulation/16-QAM2 ==
  In1 : Inport
  BitBasher : xbsIndex_r4/BitBasher  bitexpr=|  display_expr=on  sr_1=b  arith_type1=Unsigned  bin_pt1=0  sr_2=c  arith_type2=Unsigned  bin_pt2=0  sr_3=3  arith_type3=Unsigned  bin_pt3=0  sr_4=4  arith_type4=Unsigned  bin_pt4=0  dbl_ovrd=off  block_type=bitbasher
      | b={a[3:2]}
      | c={a[1:0]}
  Constant1 : xbsIndex_r4/Constant  const=-3  gui_display_data_type=Fixed-point  arith_type=Signed (2's comp)  n_bits=bitCount  bin_pt=fracLen  preci_type=Single  exp_width=8  frac_width=24  explicit_period=on  period=Ts*usedSubCar* bitPerSymb  equ=P=C  opselect=C  inp2=PCIN>>17  opr=+  inp1=P  carry=CIN  dbl_ovrd=off  block_type=constant
  Constant2 : xbsIndex_r4/Constant  const=-1  gui_display_data_type=Fixed-point  arith_type=Signed (2's comp)  n_bits=bitCount  bin_pt=fracLen  preci_type=Single  exp_width=8  frac_width=24  explicit_period=on  period=Ts*usedSubCar* bitPerSymb  equ=P=C  opselect=C  inp2=PCIN>>17  opr=+  inp1=P  carry=CIN  dbl_ovrd=off  block_type=constant
  Constant3 : xbsIndex_r4/Constant  const=3  gui_display_data_type=Fixed-point  arith_type=Signed (2's comp)  n_bits=bitCount  bin_pt=fracLen  preci_type=Single  exp_width=8  frac_width=24  explicit_period=on  period=Ts*usedSubCar* bitPerSymb  equ=P=C  opselect=C  inp2=PCIN>>17  opr=+  inp1=P  carry=CIN  dbl_ovrd=off  block_type=constant
  Constant4 : xbsIndex_r4/Constant  const=1  gui_display_data_type=Fixed-point  arith_type=Signed (2's comp)  n_bits=bitCount  bin_pt=fracLen  preci_type=Single  exp_width=8  frac_width=24  explicit_period=on  period=Ts*usedSubCar* bitPerSymb  equ=P=C  opselect=C  inp2=PCIN>>17  opr=+  inp1=P  carry=CIN  dbl_ovrd=off  block_type=constant
  Constant5 : xbsIndex_r4/Constant  const=1  gui_display_data_type=Fixed-point  arith_type=Signed (2's comp)  n_bits=bitCount  bin_pt=fracLen  preci_type=Single  exp_width=8  frac_width=24  explicit_period=on  period=Ts*usedSubCar* bitPerSymb  equ=P=C  opselect=C  inp2=PCIN>>17  opr=+  inp1=P  carry=CIN  dbl_ovrd=off  block_type=constant
  Constant6 : xbsIndex_r4/Constant  const=-3  gui_display_data_type=Fixed-point  arith_type=Signed (2's comp)  n_bits=bitCount  bin_pt=fracLen  preci_type=Single  exp_width=8  frac_width=24  explicit_period=on  period=Ts*usedSubCar* bitPerSymb  equ=P=C  opselect=C  inp2=PCIN>>17  opr=+  inp1=P  carry=CIN  dbl_ovrd=off  block_type=constant
  Constant7 : xbsIndex_r4/Constant  const=-1  gui_display_data_type=Fixed-point  arith_type=Signed (2's comp)  n_bits=bitCount  bin_pt=fracLen  preci_type=Single  exp_width=8  frac_width=24  explicit_period=on  period=Ts*usedSubCar* bitPerSymb  equ=P=C  opselect=C  inp2=PCIN>>17  opr=+  inp1=P  carry=CIN  dbl_ovrd=off  block_type=constant
  Constant9 : xbsIndex_r4/Constant  const=3  gui_display_data_type=Fixed-point  arith_type=Signed (2's comp)  n_bits=bitCount  bin_pt=fracLen  preci_type=Single  exp_width=8  frac_width=24  explicit_period=on  period=Ts*usedSubCar* bitPerSymb  equ=P=C  opselect=C  inp2=PCIN>>17  opr=+  inp1=P  carry=CIN  dbl_ovrd=off  block_type=constant
  Mux : xbsIndex_r4/Mux  inputs=4  en=off  latency=1  precision=Full  arith_type=Unsigned  n_bits=16  bin_pt=14  quantization=Truncate  overflow=Wrap  dbl_ovrd=off  block_type=mux
  Mux1 : xbsIndex_r4/Mux  inputs=4  en=off  latency=1  precision=Full  arith_type=Unsigned  n_bits=16  bin_pt=14  quantization=Truncate  overflow=Wrap  dbl_ovrd=off  block_type=mux
  Out2 : Outport
  Out3 : Outport  Port=2
  wires:
  Mux1/1 -> Out3/1
  In1/1 -> BitBasher/1
  Constant1/1 -> Mux/2
  Constant2/1 -> Mux/3
  BitBasher/1 -> Mux/1
  Constant9/1 -> Mux1/2
  Constant5/1 -> Mux1/3
  Constant7/1 -> Mux1/5
  Constant6/1 -> Mux1/4
  BitBasher/2 -> Mux1/1
  Constant4/1 -> Mux/5
  Mux/1 -> Out2/1
  Constant3/1 -> Mux/4

== system Basic_DMT/Sysgen_Modulation/16-QAM3 ==
  In1 : Inport
  BitBasher : xbsIndex_r4/BitBasher  bitexpr=|  display_expr=on  sr_1=b  arith_type1=Unsigned  bin_pt1=0  sr_2=c  arith_type2=Unsigned  bin_pt2=0  sr_3=3  arith_type3=Unsigned  bin_pt3=0  sr_4=4  arith_type4=Unsigned  bin_pt4=0  dbl_ovrd=off  block_type=bitbasher
      | b={a[3:2]}
      | c={a[1:0]}
  Constant1 : xbsIndex_r4/Constant  const=-3  gui_display_data_type=Fixed-point  arith_type=Signed (2's comp)  n_bits=bitCount  bin_pt=fracLen  preci_type=Single  exp_width=8  frac_width=24  explicit_period=on  period=Ts*usedSubCar* bitPerSymb  equ=P=C  opselect=C  inp2=PCIN>>17  opr=+  inp1=P  carry=CIN  dbl_ovrd=off  block_type=constant
  Constant2 : xbsIndex_r4/Constant  const=-1  gui_display_data_type=Fixed-point  arith_type=Signed (2's comp)  n_bits=bitCount  bin_pt=fracLen  preci_type=Single  exp_width=8  frac_width=24  explicit_period=on  period=Ts*usedSubCar* bitPerSymb  equ=P=C  opselect=C  inp2=PCIN>>17  opr=+  inp1=P  carry=CIN  dbl_ovrd=off  block_type=constant
  Constant3 : xbsIndex_r4/Constant  const=3  gui_display_data_type=Fixed-point  arith_type=Signed (2's comp)  n_bits=bitCount  bin_pt=fracLen  preci_type=Single  exp_width=8  frac_width=24  explicit_period=on  period=Ts*usedSubCar* bitPerSymb  equ=P=C  opselect=C  inp2=PCIN>>17  opr=+  inp1=P  carry=CIN  dbl_ovrd=off  block_type=constant
  Constant4 : xbsIndex_r4/Constant  const=1  gui_display_data_type=Fixed-point  arith_type=Signed (2's comp)  n_bits=bitCount  bin_pt=fracLen  preci_type=Single  exp_width=8  frac_width=24  explicit_period=on  period=Ts*usedSubCar* bitPerSymb  equ=P=C  opselect=C  inp2=PCIN>>17  opr=+  inp1=P  carry=CIN  dbl_ovrd=off  block_type=constant
  Constant5 : xbsIndex_r4/Constant  const=1  gui_display_data_type=Fixed-point  arith_type=Signed (2's comp)  n_bits=bitCount  bin_pt=fracLen  preci_type=Single  exp_width=8  frac_width=24  explicit_period=on  period=Ts*usedSubCar* bitPerSymb  equ=P=C  opselect=C  inp2=PCIN>>17  opr=+  inp1=P  carry=CIN  dbl_ovrd=off  block_type=constant
  Constant6 : xbsIndex_r4/Constant  const=-3  gui_display_data_type=Fixed-point  arith_type=Signed (2's comp)  n_bits=bitCount  bin_pt=fracLen  preci_type=Single  exp_width=8  frac_width=24  explicit_period=on  period=Ts*usedSubCar* bitPerSymb  equ=P=C  opselect=C  inp2=PCIN>>17  opr=+  inp1=P  carry=CIN  dbl_ovrd=off  block_type=constant
  Constant7 : xbsIndex_r4/Constant  const=-1  gui_display_data_type=Fixed-point  arith_type=Signed (2's comp)  n_bits=bitCount  bin_pt=fracLen  preci_type=Single  exp_width=8  frac_width=24  explicit_period=on  period=Ts*usedSubCar* bitPerSymb  equ=P=C  opselect=C  inp2=PCIN>>17  opr=+  inp1=P  carry=CIN  dbl_ovrd=off  block_type=constant
  Constant9 : xbsIndex_r4/Constant  const=3  gui_display_data_type=Fixed-point  arith_type=Signed (2's comp)  n_bits=bitCount  bin_pt=fracLen  preci_type=Single  exp_width=8  frac_width=24  explicit_period=on  period=Ts*usedSubCar* bitPerSymb  equ=P=C  opselect=C  inp2=PCIN>>17  opr=+  inp1=P  carry=CIN  dbl_ovrd=off  block_type=constant
  Mux : xbsIndex_r4/Mux  inputs=4  en=off  latency=1  precision=Full  arith_type=Unsigned  n_bits=16  bin_pt=14  quantization=Truncate  overflow=Wrap  dbl_ovrd=off  block_type=mux
  Mux1 : xbsIndex_r4/Mux  inputs=4  en=off  latency=1  precision=Full  arith_type=Unsigned  n_bits=16  bin_pt=14  quantization=Truncate  overflow=Wrap  dbl_ovrd=off  block_type=mux
  Out2 : Outport
  Out3 : Outport  Port=2
  wires:
  Mux1/1 -> Out3/1
  In1/1 -> BitBasher/1
  Constant1/1 -> Mux/2
  Constant2/1 -> Mux/3
  BitBasher/1 -> Mux/1
  Constant9/1 -> Mux1/2
  Constant5/1 -> Mux1/3
  Constant7/1 -> Mux1/5
  Constant6/1 -> Mux1/4
  BitBasher/2 -> Mux1/1
  Constant4/1 -> Mux/5
  Mux/1 -> Out2/1
  Constant3/1 -> Mux/4
